simulink model "35-Bus_Network_Electricity_Transmission_Model"  (R2023b)
settings: Solver=VariableStepAuto  StartTime=0.0  StopTime=10  RelTol=1e-3
undefined symbols (not defined in the file): D1, D11, Delta
libraries: spsSeriesRLCBranchLib x47, spsLoadFlowBusLib x35, spsThreePhaseSeriesRLCLoadLib x27, spsDistributedParametersLineLib x22, spsGenericPowerSystemStabilizerLib x20, spsThreePhaseTransformerTwoWindingsLib x19, spsThreePhaseVIMeasurementLib x13, spsSynchronousMachinepuStandardLib x10, spsExcitationSystemLib x10, spsHydraulicTurbineandGovernorLib x10, spsThreePhaseParallelRLCLoadLib x4, spsGroundLib x3
(part 1 of 7)
settings Model: Creator=3.22  LastModifiedBy=3.22

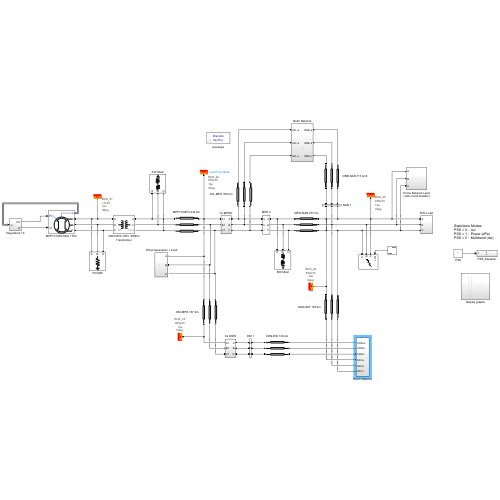
[thumbnail: Simulink's stored preview of the top-level diagram]
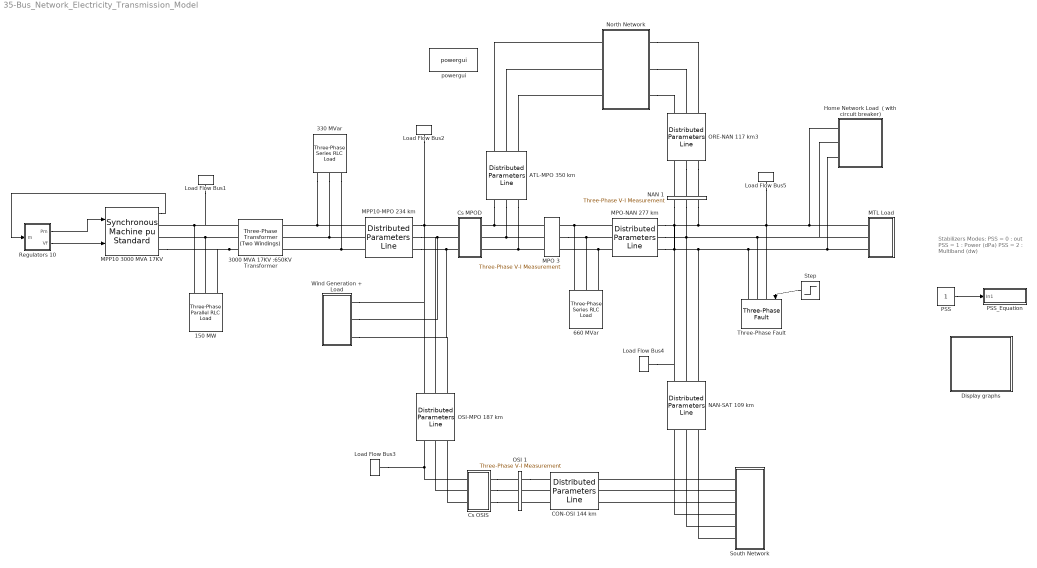
== system 35-Bus_Network_Electricity_Transmission_Model ==
  note: Stabilizers Modes:
      | PSS = 0 :  out
      | PSS = 1 :  Power (dPa)
      | PSS = 2 :  Multiband (dw)
  " Wind Generation + Load" : Subsystem
  150 MW : spsThreePhaseParallelRLCLoadLib/Three-Phase Parallel RLC Load  LConnTagsString=A|B|C  Configuration=Y (grounded)  NominalVoltage=1000  Vabc=[1e3 1e3 1e3]  Vabcp=[1e3 1e3 1e3]  NominalFrequency=60  UnbalancedPower=off  ActivePower=150e6  InductivePower=0  CapacitivePower=0  Pabc=[10e3 9e3 11e3]  QLabc=[100 90 110]  QCabc=[100 90 110]  Pabcp=[10e3 9e3 11e3]  QLabcp=[100 90 110]  QCabcp=[100 90 110]  Measurements=None  LoadType=constant Z
  "3000 MVA 17KV :650KV Transformer " : spsThreePhaseTransformerTwoWindingsLib/Three-Phase Transformer (Two Windings)  Winding1Connection=Delta (D1)  Winding2Connection=Yg  CoreType=Three single-phase transformers  SetSaturation=off  Hysteresis=off  DataFile='hysteresis'  SetInitialFlux=off  Measurements=None  UNITS=pu  NominalPower=[ 3000e6 , 60 ]  Winding1=[ 17e3 , 0.002 , 0.08 ]  Winding2=[ 650e3 , 0.002 , 0.08 ]  Rm=500  Lm=500  L0=0.5  Saturation=[ 0,0 ; 0.0024,1.2 ; 1.0,1.52 ]  InitialFluxes=[ 0.8 , -0.8 , 0.7 ]  BreakLoop=off  DiscreteSolver=Trapezoidal iterative  DataType=off  TransfoNumber=1
  330 MVar : spsThreePhaseSeriesRLCLoadLib/Three-Phase Series RLC Load  LConnTagsString=A|B|C  Configuration=Y (grounded)  NominalVoltage=1000  Vabc=[1e3 1e3 1e3]  Vabcp=[1e3 1e3 1e3]  NominalFrequency=60  UnbalancedPower=off  ActivePower=1100e3  InductivePower=330e6  CapacitivePower=0  Pabc=[10e3 9e3 11e3]  QLabc=[100 90 110]  QCabc=[100 90 110]  Pabcp=[10e3 9e3 11e3]  QLabcp=[100 90 110]  QCabcp=[100 90 110]  Measurements=None  LoadType=constant Z
  660 MVar : spsThreePhaseSeriesRLCLoadLib/Three-Phase Series RLC Load  LConnTagsString=A|B|C  Configuration=Y (grounded)  NominalVoltage=1000  Vabc=[1e3 1e3 1e3]  Vabcp=[1e3 1e3 1e3]  NominalFrequency=60  UnbalancedPower=off  ActivePower=2200e3  InductivePower=660e6  CapacitivePower=0  Pabc=[10e3 9e3 11e3]  QLabc=[100 90 110]  QCabc=[100 90 110]  Pabcp=[10e3 9e3 11e3]  QLabcp=[100 90 110]  QCabcp=[100 90 110]  Measurements=None  LoadType=constant Z
  ATL-MPO 350 km : spsDistributedParametersLineLib/Distributed Parameters Line  Phases=3  Length=350  Frequency=60  Resistance=[0.01273 0.3864]/6  Inductance="[0.9337e-3  4.1264e-3]/6"  Capacitance=[12.74e-9 7.751e-9]*6  x1=[-0.00198 6.98010668023183e-15 0.00211514985966667 -0.00384910891782008;-0.00192 6.88834857923299e-15 0.00223032100016454 -0.00383079412320694;-0.00186 6.79306627181897e-15 0.00234435106722713 -0.00381051942353543;-0.0018 6.69430850617886e-15 0.00245718172096511 -0.00378829519171654;-0.00174 6.59212580861038e-15 0.00256875523513113 -0.00376413279807792;-0.00168 6.48657045766974e-15 0.00267901452665373 -0.00373804460454662;-0.00162 6.37769645742491e-15 0.002787903184842 -0.00371004395832451;-0.00156 6.26555950982618e-15 0.00289536550024637 -0.0036801451850596;-0.0015 6.150216986208e-15 0.00300134649316061 -0.00364836358151674;-0.00144 6.03172789793673e-15 0.00310579194175044 -0.00361471540775158;-0.00138 5.91015286621936e-15 0.00320864840979444 -0.00357921787879154;-0.00132 5.78555409108856e-15 0.00330986327402298 -0.00354188915582838;-0.00126 5.65799531958002e-15 0.00340938475104129 -0.0035027483369265;-0.0012 5.52754181311824e-15 0.00350716192382279 -0.00346181544725211;-0.00114 5.39426031412764e-15 0.00360314476775915 -0.00341911142882791;-0.00108 5.25821901188587e-15 0.00369728417625386 -0.0033746581298188;-0.00102 5.1194875076369e-15 0.00378953198584605 -0.00332847829335396;-0.00096 4.97813677898177e-15 0.00387984100085178 -0.00328059554589104;-0.0009 4.83423914356512e-15 0.00396816501751025 -0.00323103438512841;-0.00084 4.68786822207615e-15 0.00405445884762251 -0.00317982016747169;-0.00078 4.53909890058292e-15 0.00413867834167054 -0.00312697909506097;-0.00072 4.38800729221925e-15 0.00422078041140498 -0.00307253820236529;-0.00066 4.23467069824383e-15 0.0043007230518899 -0.0030165253423513;-0.0006 4.07916756849147e-15 0.00437846536299324 -0.00295896917223319;-0.00054 3.92157746123672e-15 0.00445396757031214 -0.00289989913881109;-0.00048 3.76198100249039e-15 0.00452719104552221 -0.00283934546340561;-0.00042 3.60045984474976e-15 0.00459809832614052 -0.00277733912639597;-0.00036 3.43709662522371e-15 0.00466665313469209 -0.00271391185136995;-0.0003 3.27197492355395e-15 0.00473282039727011 -0.00264909608889343;-0.00024 3.10517921905415e-15 0.00479656626148042 -0.00258292499990818;-0.00018 2.93679484748877e-15 0.00485785811376101 -0.002515432438766;-0.00012 2.76690795741369e-15 0.0049166645960677 -0.0024466529359083;-6e-05 2.59560546610101e-15 0.00497295562191752 -0.00237662168019965]  x2=[-0.00198 9.14273446462953e-13 -0.141743524193211 -0.279232793755801;-0.00192 9.90097800622471e-13 -0.134363025534958 -0.282492907357275;-0.00186 1.06541560245229e-12 -0.126913784270099 -0.285608492367477;-0.0018 1.14018831797327e-12 -0.119399611568109 -0.288577954795545;-0.00174 1.21437769208252e-12 -0.11182435181859 -0.291399775409632;-0.00168 1.28794576812539e-12 -0.104191880664404 -0.294072510514171;-0.00162 1.36085490731478e-12 -0.0965061030188257 -0.296594792688496;-0.00156 1.43306780798787e-12 -0.0887709510677152 -0.29896533148644;-0.0015 1.50454752469036e-12 -0.0809903822577399 -0.301182914096551;-0.00144 1.57525748707837e-12 -0.0731683772716712 -0.30324640596259;-0.00138 1.64516151862858e-12 -0.0653089379917943 -0.305154751363989;-0.00132 1.71422385514677e-12 -0.0574160854524703 -0.306906973955978;-0.00126 1.78240916306545e-12 -0.0494938577829015 -0.308502177269103;-0.0012 1.84968255752117e-12 -0.0415463081411497 -0.309939545167873;-0.00114 1.91600962020226e-12 -0.0335775026404654 -0.31121834226831;-0.00108 1.98135641695787e-12 -0.0255915182689893 -0.312337914314189;-0.00102 2.0456895151593e-12 -0.0175924408038899 -0.313297688511763;-0.00096 2.10897600080479e-12 -0.00958436272100424 -0.31409717382282;-0.0009 2.17118349535886e-12 -0.0015713811010519 -0.3147359612159;-0.00084 2.23228017231786e-12 0.00644240446650752 -0.31521372387557;-0.00078 2.29223477349289e-12 0.0144528939809 -0.315530217369625;-0.00072 2.35101662500219e-12 0.0224559891276729 -0.315685279774147;-0.00066 2.40859565296433e-12 0.0304475953754693 -0.315678831756342;-0.0006 2.46494239888469e-12 0.0384236240708646 -0.315510876615137;-0.00054 2.52002803472689e-12 0.0463799945301984 -0.315181500279485;-0.00048 2.57382437766175e-12 0.0543126361273268 -0.314690871264405;-0.00042 2.62630390448619e-12 0.0622174903762302 -0.314039240584767;-0.00036 2.67743976570459e-12 0.0700905130074102 -0.313226941626869;-0.0003 2.72720579926545e-12 0.0779276760370118 -0.312254389977866;-0.00024 2.77557654394643e-12 0.085724969827615 -0.311122083213152;-0.00018 2.82252725238078e-12 0.093478405139639 -0.309830600641792;-0.00012 2.8680339037185e-12 0.101184015172311 -0.308380603010131;-6e-05 2.91207321591591e-12 0.108837857593156 -0.306772832163753]  x3=[-0.00198 -3.31408931648922e-14 -0.0161917965503002 0.00683182870242155;-0.00192 -3.27443580437374e-14 -0.0163349113753115 0.00651312629500997;-0.00186 -3.23310703039613e-14 -0.0164696689578288 0.00619109165183713;-0.0018 -3.19012413912081e-14 -0.0165960003533827 0.00586588953177699;-0.00174 -3.14550912138921e-14 -0.0167138409284971 0.00553768631424321;-0.00168 -3.09928480306878e-14 -0.0168231303937561 0.00520664991406639;-0.00162 -3.05147483337489e-14 -0.01692381283465 0.00487294969558571;-0.00156 -3.00210367277148e-14 -0.0170158367401816 0.004536756385999;-0.0015 -2.95119658045659e-14 -0.0170991550292203 0.0041982419880156;-0.00144 -2.89877960143928e-14 -0.0171737250745901 0.00385757969185654;-0.00138 -2.8448795532146e-14 -0.0172395087248778 0.00351494378664725;-0.00132 -2.78952401204316e-14 -0.0172964723239523 0.00317050957124801;-0.00126 -2.73274129884268e-14 -0.0173445867281838 0.00282445326456784;-0.0012 -2.67456046469846e-14 -0.0173838273213541 0.00247695191540763;-0.00114 -2.6150112760003e-14 -0.0174141740272506 0.00212818331187868;-0.00108 -2.55412419921349e-14 -0.0174356113199377 0.00177832589044307;-0.00102 -2.49193038529158e-14 -0.0174481282317006 0.00142755864462222;-0.00096 -2.42846165373897e-14 -0.0174517183586558 0.00107606103342054;-0.0009 -2.36375047633149e-14 -0.017446379864028 0.000724012889510833;-0.00084 -2.29782996050323e-14 -0.0174321154790897 0.000371594327228634;-0.00078 -2.23073383240817e-14 -0.0174089325017639 1.89856504223522e-05;-0.00072 -2.16249641966523e-14 -0.0173768427928901 -0.000333632739793501;-0.00066 -2.09315263379564e-14 -0.0173358627701563 -0.000686080437334852;-0.0006 -2.02273795236159e-14 -0.0172860133996994 -0.00103817712344715;-0.00054 -1.95128840081521e-14 -0.0172273201853784 -0.00138974265895979;-0.00048 -1.87884053406732e-14 -0.0171598131557262 -0.00174059717644861;-0.00042 -1.80543141778521e-14 -0.0170835268485868 -0.00209056117225943;-0.00036 -1.73109860942922e-14 -0.0169985002934443 -0.00243945559834538;-0.0003 -1.65588013903763e-14 -0.0169047769914555 -0.00278710195387127;-0.00024 -1.57981448976976e-14 -0.0168024048931935 -0.00313332237653783;-0.00018 -1.50294057821731e-14 -0.0166914363741154 -0.00347793973357942;-0.00012 -1.42529773449389e-14 -0.016571928207766 -0.00382077771238837;-6e-05 -1.34692568211303e-14 -0.0164439415367315 -0.0041616609107198]  x4=[-0.00198 2.98411089605461e-14 0.0114570231609346 -0.0122817125842966;-0.00192 3.00466879551929e-14 0.0117485485103798 -0.0120667412107585;-0.00186 3.02368945090828e-14 0.0120340630853189 -0.0118455962694493;-0.0018 3.04116313090283e-14 0.0123134208112197 -0.0116183909022071;-0.00174 3.05708089564538e-14 0.0125864787635076 -0.0113852413514962;-0.00168 3.07143460131335e-14 0.0128530972406887 -0.0111462669009348;-0.00162 3.08421690428571e-14 0.0131131398358235 -0.0109015898142675;-0.00156 3.09542126490005e-14 0.0133664735063153 -0.010651335272813;-0.0015 3.10504195079847e-14 0.0136129686419773 -0.010395631311419;-0.00144 3.11307403986028e-14 0.0138524991313433 -0.0101346087529568;-0.00138 3.1195134227203e-14 0.014084942426189 -0.00986840114139055;-0.00132 3.12435680487128e-14 0.0143101796042296 -0.00959714467345329;-0.00126 3.12760170834941e-14 0.014528095429963 -0.00932097812896625;-0.0012 3.12924647300211e-14 0.014738578413626 -0.00904004279983656;-0.00114 3.1292902573374e-14 0.0149415208682351 -0.00875448241776969;-0.00108 3.1277330389544e-14 0.0151368189646803 -0.00846444308073365;-0.00102 3.12457561455481e-14 0.015324372784847 -0.00817007317821258;-0.00096 3.11981959953529e-14 0.0155040863727352 -0.00787152331528794;-0.0009 3.11346742716102e-14 0.0156758677835524 -0.00756894623558618;-0.00084 3.10552234732074e-14 0.0158396291307549 -0.00726249674313224;-0.00078 3.09598842486412e-14 0.0159952866310113 -0.00695233162314901;-0.00072 3.08487053752205e-14 0.0161427606470684 -0.00663860956184305;-0.00066 3.07217437341113e-14 0.0162819757284946 -0.00632149106521786;-0.0006 3.05790642812352e-14 0.0164128606502817 -0.00600113837695597;-0.00054 3.04207400140367e-14 0.0165353484492854 -0.00567771539541215;-0.00048 3.02468519341363e-14 0.0166493764584843 -0.00535138758975991;-0.00042 3.00574890058889e-14 0.0167548863390419 -0.00502232191533449;-0.00036 2.98527481108675e-14 0.0168518241101538 -0.00469068672821533;-0.0003 2.96327339982972e-14 0.016940140176665 -0.0043566516990921;-0.00024 2.93975592314635e-14 0.0170197893544441 -0.00402038772645795;-0.00018 2.91473441301224e-14 0.0170907308934998 -0.00368206684917471;-0.00012 2.88822167089435e-14 0.0171529284988301 -0.00334186215845466;-6e-05 2.86023126120142e-14 0.0172063503489906 -0.00299994770930384]  x5=0.0019793954844851  V1=[4.219e-16 0.0001256 0.0001256;377 377 377;2.896 1.02 -0.5506]  V2=[3.447e-16 8.016e-05 8.016e-05;377 377 377;2.788 1.015 -0.5555]  I1=[4.128e-19 5.188e-07 5.188e-07;377 377 377;2.697 1.572 0.0007381]  I2=[5.884e-19 5.436e-07 5.436e-07;377 377 377;2.289 0.05248 -1.518]  nHarmo=1  Measurements=None  Decoupling=off  VsMag0=0  VrMag0=0  VsAngle0=0  VrAngle0=0  IsMag0=0  IrMag0=0  IsAngle0=0  IrAngle0=0
      settings: LibrarySourceBlock=sps_lib/Power Grid Elements/Distributed Parameters Line
  CON-OSI 144 km : spsDistributedParametersLineLib/Distributed Parameters Line  Phases=3  Length=144  Frequency=60  Resistance=[0.01273 0.3864]/6  Inductance="[0.9337e-3  4.1264e-3]/6"  Capacitance=[12.74e-9 7.751e-9]*6  x1=[-0.00084 -6.12106331906545e-12 0 0;-0.00078 -5.96931950471425e-12 0 0;-0.00072 -5.8145216762041e-12 0 0;-0.00066 -5.65674903096439e-12 0 0;-0.0006 -5.49608228839574e-12 0 0;-0.00054 -5.33260364857242e-12 -13.3263292704613 8.49263982125866;-0.00048 -5.1663967501873e-12 -13.5399966121397 8.3110034847415;-0.00042 -4.99754662776075e-12 -13.7467366413609 8.12511508527185;-0.00036 -4.8261396681354e-12 -13.9464435861059 7.93506972678971;-0.0003 -4.65226356627902e-12 -14.1390152726117 7.74096464001211;-0.00024 -4.47600728041818e-12 -14.324353177645 7.54289913268811;-0.00018 -4.29746098652558e-12 -14.5023624789089 7.34097453879107;-0.00012 -4.11671603218432e-12 -14.6729521035559 7.13529416667437;-6e-05 -3.93386488985283e-12 -14.8360347747817 6.92596324621692]  x2=[-0.00084 -4.40472411926851e-12 0 0;-0.00078 -4.29950048512916e-12 0 0;-0.00072 -4.19207714709598e-12 0 0;-0.00066 -4.08250906493367e-12 0 0;-0.0006 -3.97085229569764e-12 0 0;-0.00054 -3.85716396505422e-12 -8.94549366124329 5.71026905715697;-0.00048 -3.74150223805408e-12 -9.08922753957406 5.58838070697636;-0.00042 -3.62392628937395e-12 -9.22831120114597 5.46363323796466;-0.00036 -3.50449627304171e-12 -9.36267348818779 5.33609047323209;-0.0003 -3.38327329166053e-12 -9.49224565847074 5.20581766601379;-0.00024 -3.26031936514764e-12 -9.61696142047828 5.07288146628511;-0.00018 -3.13569739900377e-12 -9.73675696732208 4.93734988666221;-0.00012 -3.00947115212954e-12 -9.85157100938683 4.79929226760556;-6e-05 -2.88170520420524e-12 -9.96134480568707 4.65877924194407]  x3=[-0.00084 5.02734058306821e-15 0 0;-0.00078 6.70201184862852e-15 0 0;-0.00072 8.37325424108812e-15 0 0;-0.00066 1.0040212721958e-14 0 0;-0.0006 1.17020344444776e-14 0 0;-0.00054 1.33578691899466e-14 -0.627617797454106 -0.11745005126189;-0.00048 1.50068698027131e-14 -0.620824228506745 -0.128185682906486;-0.00042 1.66481926235933e-14 -0.613713034412567 -0.138855732387108;-0.00036 1.82809979215042e-14 -0.60628785338987 -0.149454740709282;-0.0003 1.99044503230843e-14 -0.598552484298468 -0.159977285224503;-0.00024 2.15177192400873e-14 -0.59051088469612 -0.170417982404563;-0.00018 2.31199792943252e-14 -0.582167168813775 -0.180771490595862;-0.00012 2.47104107399481e-14 -0.573525605450653 -0.191032512752299;-6e-05 2.62881998828405e-14 -0.564590615790247 -0.201195799145338]  x4=[-0.00084 -1.00461865876865e-13 0 0;-0.00078 -1.00433753021638e-13 0 0;-0.00072 -1.00354256402562e-13 0 0;-0.00066 -1.00223416691577e-13 0 0;-0.0006 -1.00041300828697e-13 0 0;-0.00054 -9.98080019877624e-14 0.169804112382748 0.458131219894259;-0.00048 -9.95236395287709e-14 0.15407641971246 0.462833113851965;-0.00042 -9.91883589368111e-14 0.138269898698842 0.467298213836452;-0.00036 -9.8802331747629e-14 0.122392636250115 0.471524235420061;-0.0003 -9.83657554598677e-14 0.106452755467127 0.475509016492064;-0.00024 -9.78788534340229e-14 0.0904584114874216 0.479250518364833;-0.00018 -9.73418747781681e-14 0.0744177873129197 0.482746826816875;-0.00012 -9.67550942205056e-14 0.0583390896233459 0.485996153072182;-6e-05 -9.61188119688114e-14 0.0422305445775383 0.488996834715401]  x5=0.000814379856473869  V1=[3.066e-13 0.3294 0.3294;377 377 377;-0.5534 -1.851 2.861]  V2=[2.167e-13 0.2213 0.2213;377 377 377;-0.5727 -1.852 2.86]  I1=[4.19e-16 0.002316 0.002316;377 377 377;0.2564 -0.79 -2.361]  I2=[5.677e-16 0.002387 0.002387;377 377 377;-1.374 -3.038 1.674]  nHarmo=1  Measurements=None  Decoupling=off  VsMag0=0  VrMag0=0  VsAngle0=0  VrAngle0=0  IsMag0=0  IrMag0=0  IsAngle0=0  IrAngle0=0
      settings: LibrarySourceBlock=sps_lib/Power Grid Elements/Distributed Parameters Line
  Cs MPOD : Subsystem
  Cs OSIS : Subsystem
  Display graphs : Subsystem
  Home Network Load （with circuit breaker) : Subsystem
  Load Flow Bus1 : spsLoadFlowBusLib/Load Flow Bus  LConnTagsString=a  Phases=single  Connectors=on one side  ID=BUS_21  Vbase=17e3  Vref=1  Vangle=0  VLF=1  VLFb=1  VLFc=1  angleLF=0  angleLFb=0  angleLFc=0
  Load Flow Bus2 : spsLoadFlowBusLib/Load Flow Bus  LConnTagsString=a  Phases=single  Connectors=on one side  ID=BUS_22  Vbase=650e3  Vref=1  Vangle=0  VLF=1  VLFb=1  VLFc=1  angleLF=0  angleLFb=0  angleLFc=0
  Load Flow Bus3 : spsLoadFlowBusLib/Load Flow Bus  LConnTagsString=a  Phases=single  Connectors=on one side  ID=BUS_23  Vbase=650e3  Vref=1  Vangle=0  VLF=1  VLFb=1  VLFc=1  angleLF=0  angleLFb=0  angleLFc=0
  Load Flow Bus4 : spsLoadFlowBusLib/Load Flow Bus  LConnTagsString=a  Phases=single  Connectors=on one side  ID=BUS_24  Vbase=650e3  Vref=1  Vangle=0  VLF=1  VLFb=1  VLFc=1  angleLF=0  angleLFb=0  angleLFc=0
  Load Flow Bus5 : spsLoadFlowBusLib/Load Flow Bus  LConnTagsString=a  Phases=single  Connectors=on one side  ID=BUS_25  Vbase=650e3  Vref=1  Vangle=0  VLF=1  VLFb=1  VLFc=1  angleLF=0  angleLFb=0  angleLFc=0
  MPO 3 : spsThreePhaseVIMeasurementLib/Three-Phase V-I Measurement  VoltageMeasurement=no  SetLabelV=off  LabelV=Vabc_MPO3  Vpu=off  VpuLL=off  CurrentMeasurement=no  SetLabelI=off  LabelI=Iabc  Ipu=off  Pbase=100e6  Vbase=500e3  OutputType=Complex  PhasorSimulation=off  PSBequivalent=0
  MPO-NAN 277 km : spsDistributedParametersLineLib/Distributed Parameters Line  Phases=3  Length=277  Frequency=60  Resistance=[0.01273 0.3864]/6  Inductance="[0.9337e-3  4.1264e-3]/6"  Capacitance=[12.74e-9 7.751e-9]*6  x1=[-0.00162 6.37769645742491e-15 0.002787903184842 -0.00371004395832451;-0.00156 6.26555950982618e-15 0.00289536550024637 -0.0036801451850596;-0.0015 6.150216986208e-15 0.00300134649316061 -0.00364836358151674;-0.00144 6.03172789793673e-15 0.00310579194175044 -0.00361471540775158;-0.00138 5.91015286621936e-15 0.00320864840979444 -0.00357921787879154;-0.00132 5.78555409108856e-15 0.00330986327402298 -0.00354188915582838;-0.00126 5.65799531958002e-15 0.00340938475104129 -0.0035027483369265;-0.0012 5.52754181311824e-15 0.00350716192382279 -0.00346181544725211;-0.00114 5.39426031412764e-15 0.00360314476775915 -0.00341911142882791;-0.00108 5.25821901188587e-15 0.00369728417625386 -0.0033746581298188;-0.00102 5.1194875076369e-15 0.00378953198584605 -0.00332847829335396;-0.00096 4.97813677898177e-15 0.00387984100085178 -0.00328059554589104;-0.0009 4.83423914356512e-15 0.00396816501751025 -0.00323103438512841;-0.00084 4.68786822207615e-15 0.00405445884762251 -0.00317982016747169;-0.00078 4.53909890058292e-15 0.00413867834167054 -0.00312697909506097;-0.00072 4.38800729221925e-15 0.00422078041140498 -0.00307253820236529;-0.00066 4.23467069824383e-15 0.0043007230518899 -0.0030165253423513;-0.0006 4.07916756849147e-15 0.00437846536299324 -0.00295896917223319;-0.00054 3.92157746123672e-15 0.00445396757031214 -0.00289989913881109;-0.00048 3.76198100249039e-15 0.00452719104552221 -0.00283934546340561;-0.00042 3.60045984474976e-15 0.00459809832614052 -0.00277733912639597;-0.00036 3.43709662522371e-15 0.00466665313469209 -0.00271391185136995;-0.0003 3.27197492355395e-15 0.00473282039727011 -0.00264909608889343;-0.00024 3.10517921905415e-15 0.00479656626148042 -0.00258292499990818;-0.00018 2.93679484748877e-15 0.00485785811376101 -0.002515432438766;-0.00012 2.76690795741369e-15 0.0049166645960677 -0.0024466529359083;-6e-05 2.59560546610101e-15 0.00497295562191752 -0.00237662168019965]  x2=[-0.00162 3.45357352044025e-13 -0.0116853448372484 -0.0542657161926271;-0.00156 2.87134243606378e-13 -0.0102864722355918 -0.0545635202751054;-0.0015 2.28764231984071e-13 -0.00888233688466737 -0.054833408652393;-0.00144 1.70277180353604e-13 -0.00747365716606598 -0.0550752432446092;-0.00138 1.11703011771307e-13 -0.00606115378636113 -0.0552889003247079;-0.00132 5.30716938641543e-14 -0.00464554940838193 -0.0554742705817792;-0.00126 -5.58677650223161e-15 -0.00322756828148552 -0.055631259176974;-0.0012 -6.42423885705273e-14 -0.0018079358710177 -0.0557597857920265;-0.00114 -1.22865133045767e-13 -0.000387378487151455 -0.0558597846703454;-0.00108 -1.81425017448655e-13 0.00103337708670675 -0.0559312046506569;-0.00102 -2.39892081460267e-13 0.00245360396575279 -0.0559740091931792;-0.00096 -2.98236412250307e-13 0.00387257553567255 -0.0559881763983175;-0.0009 -3.56428159781065e-13 0.00528956582439131 -0.0559736990178678;-0.00084 -4.14437552079244e-13 0.00670384987349436 -0.0559305844587256;-0.00078 -4.72234910467854e-13 0.00811470410912923 -0.055858854779096;-0.00072 -5.2979066475037e-13 0.00952140671219937 -0.0557585466772083;-0.00066 -5.87075368339395e-13 0.0109232379876602 -0.0556297114725412;-0.0006 -6.44059713322071e-13 0.0123194807327283 -0.0554724150795658;-0.00054 -7.00714545454557e-13 0.0137094206038157 -0.0552867379740233;-0.00048 -7.57010879077872e-13 0.0150923464820012 -0.0550727751517519;-0.00042 -8.12919911947498e-13 0.0164675508368521 -0.0548306360800849;-0.00036 -8.68413039969138e-13 0.0178343300884094 -0.0545604446418457;-0.0003 -9.23461871833103e-13 0.019191984967153 -0.0542623390719667;-0.00024 -9.78038243539824e-13 0.0205398208717603 -0.0539364718867656;-0.00018 -1.03211423280908e-12 0.0218771482244773 -0.0535830098059159;-0.00012 -1.08566217336556e-12 0.0232032828239195 -0.0532021336671493;-6e-05 -1.13865466909341e-12 0.0245175461951216 -0.0527940383337362]  x3=[-0.00162 3.43834216329146e-14 -0.0035424404892329 0.000742255688742989;-0.00156 3.43011259819442e-14 -0.00355650736100562 0.000670266158361229;-0.0015 3.42012812411094e-14 -0.00356875465789576 0.000597933707427756;-0.00144 3.40839384928247e-14 -0.00357917611395991 0.000525295342561018;-0.00138 3.39491577718082e-14 -0.00358776639738859 0.000452388226890684;-0.00132 3.37970080343674e-14 -0.00359452111323406 0.0003792496610443;-0.00126 3.36275671231193e-14 -0.0035994368056589 0.000305917064063598;-0.0012 3.34409217271651e-14 -0.00360251095970401 0.000232427954260223;-0.00114 3.3237167337738e-14 -0.00360374200257538 0.000158819930020674;-0.00108 3.30164081993487e-14 -0.00360312930444875 8.51306505702711e-05;-0.00102 3.27787572564515e-14 -0.00360067317879178 1.13978167060029e-05;-0.00096 3.25243360956602e-14 -0.00359637488220375 -6.23408484918991e-05;-0.0009 3.22532748835416e-14 -0.00359023661377262 -0.000136047618959787;-0.00084 3.19657123000207e-14 -0.00358226151394994 -0.000209684784951943;-0.00078 3.16617954674286e-14 -0.00357245366294414 -0.000283214672333589;-0.00072 3.13416798752327e-14 -0.00356081807863303 -0.000356599661855663;-0.00066 3.10055293004849e-14 -0.00354736071399653 -0.000429802208401528;-0.0006 3.06535157240307e-14 -0.00353208845407106 -0.000502784860195743;-0.00054 3.02858192425202e-14 -0.003515009112427 -0.000575510277965086;-0.00048 2.99026279762677e-14 -0.00349613142717112 -0.000647941254042015;-0.00042 2.95041379730054e-14 -0.00347546505647602 -0.000720040731400798;-0.00036 2.90905531075824e-14 -0.00345302057363882 -0.000791771822616573;-0.0003 2.8662084977658e-14 -0.00342880946167165 -0.000863097828737637;-0.00024 2.82189527954445e-14 -0.00340284410742679 -0.000933982258061304;-0.00018 2.77613832755546e-14 -0.00337513779525923 -0.00100438884480374;-0.00012 2.72896105190095e-14 -0.00334570470023024 -0.0010742815676542;-6e-05 2.68038758934689e-14 -0.0033145598808551 -0.00114362466820421]  x4=[-0.00162 -2.58146661290416e-14 0.00308060475276878 -0.00196444936876967;-0.00156 -2.61439083122915e-14 0.00312699034413802 -0.00190360844875017;-0.0015 -2.6459774788965e-14 0.00317177610946707 -0.00184179360747365;-0.00144 -2.67621039559361e-14 0.00321493913553082 -0.00177903647055511;-0.00138 -2.70507411360165e-14 0.0032564573393276 -0.00171536914570542;-0.00132 -2.73255386570914e-14 0.00329630947937716 -0.00165082420630441;-0.00126 -2.75863559276715e-14 0.00333447516658827 -0.00158543467473573;-0.0012 -2.78330595088218e-14 0.00337093487469015 -0.001519234005492;-0.00114 -2.80655231824315e-14 0.00340566995022241 -0.00145225606805883;-0.00108 -2.82836280157899e-14 0.0034386626220786 -0.00138453512958664;-0.00102 -2.8487262422434e-14 0.00346989601059815 -0.00131610583735889;-0.00096 -2.86763222192387e-14 0.00349935413620237 -0.0012470032010659;-0.0009 -2.88507106797186e-14 0.00352702192756989 -0.00117726257489328;-0.00084 -2.90103385835148e-14 0.00355288522934738 -0.00110691963943403;-0.00078 -2.91551242620423e-14 0.00357693080939177 -0.00103601038343372;-0.00072 -2.92849936402726e-14 0.00359914636554 -0.000964571085377981;-0.00066 -2.93998802746321e-14 0.00361952053190303 -0.000892638294931735;-0.0006 -2.94997253869958e-14 0.0036380428846809 -0.000820248814239743;-0.00054 -2.95844778947591e-14 0.00365470394749565 -0.00074743967909793;-0.00048 -2.96540944369733e-14 0.00366949519623971 -0.000674248140005193;-0.00042 -2.97085393965288e-14 0.00368240906343689 -0.000600711643105357;-0.00036 -2.97477849183784e-14 0.00369343894211412 -0.000526867811029033;-0.0003 -2.97718109237878e-14 0.00370257918918167 -0.000452754423645189;-0.00024 -2.97806051206089e-14 0.00370982512832023 -0.000378409398732268;-0.00018 -2.97741630095679e-14 0.00371517305237345 -0.000303870772578754;-0.00012 -2.9752487886568e-14 0.00371862022524458 -0.000229176680523103;-6e-05 -2.97155908410025e-14 0.00372016488329627 -0.000154365337442997]  x5=0.00156655014057821  V1=[4.219e-16 0.0001256 0.0001256;377 377 377;3.052 1.115 -0.4557]  V2=[4.095e-15 0.006804 0.006804;377 377 377;-1.109 1.061 -0.5096]  I1=[9.849e-18 6.958e-05 6.958e-05;377 377 377;-2.423 -0.4689 -2.04]  I2=[7.867e-18 6.871e-05 6.871e-05;377 377 377;0.191 2.298 0.7273]  nHarmo=1  Measurements=None  Decoupling=off  VsMag0=0  VrMag0=0  VsAngle0=0  VrAngle0=0  IsMag0=0  IrMag0=0  IsAngle0=0  IrAngle0=0
      settings: LibrarySourceBlock=sps_lib/Power Grid Elements/Distributed Parameters Line
  MPP10 3000 MVA 17KV : spsSynchronousMachinepuStandardLib/Synchronous Machine pu Standard  PresetModel=No  MechanicalLoad=Mechanical power Pm  ShowDetailedParameters=on  RotorType=Salient-pole  Units=per unit standard parameters  MeasurementBus=off  NominalParameters="[3000e6  17000   60]"  Reactances1=[ 1.81, 0.3, 0.23, 1.76, 0.65, 0.25, 0.15 ]  Reactances2=[2.24 0.17 0.12 1.02 0.13 0.08]  dAxisTimeConstants=Short-circuit  qAxisTimeConstants=Open-circuit  TimeConstants1="[ 4.4849  0.0681  0.1  ]"  TimeConstants2=[ 8.0, 0.03, 1.0, 0.07 ]  TimeConstants3="[  4.49  0.0681  0.0513  ]"  TimeConstants4=[ 8.0, 0.03, 0.3371, 0.0295 ]  TimeConstants5=[ 1.01, 0.053, 0.1 ]  TimeConstants6=[ 1.3201, 0.023, 1.0, 0.07 ]  TimeConstants7=[0.012 0.003 0.003]  TimeConstants8=[ 1.3201, 0.0231, 0.3371, 0.0295 ]  StatorResistance=0.037875  Mechanical=[3.8 0 28]  PolePairs=20  InitialConditions=[ 0 -107.876 0.604539 0.604539 0.604539 -42.1129 -162.113 77.8871 1.28555 ]  SetSaturation=off  Saturation=[0.6404,0.7127,0.8441,0.9214,0.9956,1.082,1.19,1.316,1.457;0.7,0.7698,0.8872,0.9466,0.9969,1.046,1.1,1.151,1.201]  LoadFlowParameters=[1,0,0,0,0]  TsPowergui=0  TsBlock=-1  IterativeModel=Trapezoidal non iterative  IterativeDiscreteModel=Trapezoidal non iterative  BusType=PV  Pref=2300e6  Qref=0  Qmin=-inf  Qmax=inf  PLF=0  QLF=0
  MPP10-MPO 234 km : spsDistributedParametersLineLib/Distributed Parameters Line  Phases=3  Length=234  Frequency=60  Resistance=[0.01273 0.3864]/6  Inductance="[0.9337e-3  4.1264e-3]/6"  Capacitance=[12.74e-9 7.751e-9]*6  x1=[-0.00138 2.70565629857601e-11 1.07097252173756 -3.44845409203551;-0.00132 2.64632447283607e-11 1.18045735649416 -3.4524056782375;-0.00126 2.58563873859737e-11 1.28933824745482 -3.45459094990138;-0.0012 2.52363014380289e-11 1.39755948914386 -3.45500878900179;-0.00114 2.46033041319553e-11 1.50506571357432 -3.45365898176453;-0.00108 2.39577193208709e-11 1.6118019185753 -3.45054221877591;-0.00102 2.32998772978942e-11 1.71771349593207 -3.44566009462948;-0.00096 2.26301146271597e-11 1.82274625932461 -3.43901510711016;-0.0009 2.19487739716255e-11 1.92684647205041 -3.43061065591635;-0.00084 2.12562039177606e-11 2.02996087451708 -3.42045104092057;-0.00078 2.0552758797202e-11 2.13203671149098 -3.40854145996959;-0.00072 1.98387985054714e-11 2.23302175908777 -3.39488800622509;-0.00066 1.91146883178466e-11 2.33286435149112 -3.37949766504629;-0.0006 1.83807987024795e-11 2.43151340738587 -3.3623783104161;-0.00054 1.76375051308581e-11 2.52891845609219 -3.34353870091271;-0.00048 1.68851878857082e-11 2.62502966338734 -3.32298847522843;-0.00042 1.61242318664335e-11 2.71979785700173 -3.30073814723846;-0.00036 1.53550263921944e-11 2.81317455177639 -3.27679910062174;-0.0003 1.45779650027248e-11 2.90511197446887 -3.25118358303685;-0.00024 1.379344525699e-11 2.99556308819492 -3.22390469985591;-0.00018 1.30018685297881e-11 3.0844816164934 -3.19497640745962;-0.00012 1.22036398063995e-11 3.17182206700222 -3.16441350609689;-6e-05 1.13991674753886e-11 3.25753975473303 -3.13223163231281]  x2=[-0.00138 -8.65543103929743e-12 -11.3616240421163 12.4769698760863;-0.00132 -8.50200366804866e-12 -11.7143796266815 12.3441892266905;-0.00126 -8.34422651462434e-12 -12.061141918173 12.2050930619919;-0.0012 -8.18218030073156e-12 -12.4017335065948 12.0597525461585;-0.00114 -8.01594793220763e-12 -12.7359801389969 11.908242038084;-0.00108 -7.84561445660388e-12 -13.0637108086261 11.7506390533438;-0.00102 -7.67126701967385e-12 -13.384757842416 11.587024224537;-0.00096 -7.49299482078784e-12 -13.6989569867718 11.4174812600333;-0.0009 -7.31088906729689e-12 -14.0061474916055 11.2420969011463;-0.00084 -7.12504292786941e-12 -14.3061721925787 11.0609608777545;-0.00078 -6.93555148482438e-12 -14.5988775915105 10.8741658623946;-0.00072 -6.74251168548546e-12 -14.8841139349102 10.6818074228481;-0.00066 -6.54602229258095e-12 -15.1617352905941 10.4839839732469;-0.0006 -6.34618383371497e-12 -15.4315996223466 10.2807967237232;-0.00054 -6.14309854993566e-12 -15.6935688625891 10.0723496286284;-0.00048 -5.9368703434268e-12 -15.9475089830177 9.85874933334797;-0.00042 -5.7276047243495e-12 -16.1932900631746 9.64010511973986;-0.00036 -5.51540875686124e-12 -16.4307863569175 9.41652885022383;-0.0003 -5.30039100433995e-12 -16.6598763567542 9.18813491055058;-0.00024 -5.08266147384086e-12 -16.8804428560076 8.95504015127987;-0.00018 -4.86233155981498e-12 -17.0923730087812 8.71736382799765;-0.00012 -4.63951398711753e-12 -17.2955583876928 8.47522754030267;-6e-05 -4.41432275333592e-12 -17.4898950393481 8.22875516959387]  x3=[-0.00138 -3.72430274266343e-13 1.48681909924038 0.371734732614772;-0.00132 -3.85202426918902e-13 1.46705787960671 0.397412025036263;-0.00126 -3.97777502892126e-13 1.44654608605372 0.422885994122415;-0.0012 -4.10149068544788e-13 1.425294212794 0.448143606919939;-0.00114 -4.22310794355298e-13 1.40331313267862 0.473171941167422;-0.00108 -4.34256458160011e-13 1.3806140916343 0.497958191906591;-0.00102 -4.45979948336592e-13 1.3572087029099 0.522489678033571;-0.00096 -4.57475266930842e-13 1.33310894113475 0.54675384878677;-0.0009 -4.68736532725359e-13 1.30832713619229 0.570738290168081;-0.00084 -4.79757984248478e-13 1.28287596691186 0.59443073129411;-0.00078 -4.90533982721948e-13 1.25676845458192 0.617819050674192;-0.00072 -5.01059014945832e-13 1.23001795628822 0.640891282411966;-0.00066 -5.11327696119163e-13 1.20263815807995 0.663635622327348;-0.0006 -5.2133477259491e-13 1.17464306796782 0.686040433995771;-0.00054 -5.31075124567838e-13 1.14604700875721 0.708094254701593;-0.00048 -5.40543768693897e-13 1.1168646107204 0.729785801302631;-0.00042 -5.49735860639793e-13 1.08711080411146 0.751103976002832;-0.00036 -5.58646697561434e-13 1.05680081152764 0.772037872030105;-0.0003 -5.67271720509998e-13 1.02595014012121 0.792576779216427;-0.00024 -5.75606516764374e-13 0.994574573665711 0.812710189477367;-0.00018 -5.83646822088787e-13 0.962690164480702 0.832427802188212;-0.00012 -5.91388522914467e-13 0.930313225219076 0.851719529453961;-6e-05 -5.98827658444219e-13 0.897460320521216 0.870575501270474]  x4=[-0.00138 5.47927057792979e-13 -1.67626482985383 -0.1532069712362;-0.00132 5.58217241869159e-13 -1.66264653750453 -0.181204688115209;-0.00126 5.68221831689729e-13 -1.64817760446446 -0.2091096973275;-0.0012 5.77935708721675e-13 -1.63286543330713 -0.236907722154735;-0.00114 5.87353903166015e-13 -1.61671785802224 -0.264584540613765;-0.00108 5.96471596500443e-13 -1.59974314000767 -0.292125992732857;-0.00102 6.05284123944573e-13 -1.58194996384282 -0.319517987796198;-0.00096 6.13786976846528e-13 -1.56334743284539 -0.34674651155297;-0.0009 6.2197580498965e-13 -1.54394506441398 -0.373797633387292;-0.00084 6.29846418818147e-13 -1.52375278515879 -0.400657513445387;-0.00078 6.37394791580554e-13 -1.502780925823 -0.427312409716304;-0.00072 6.44617061389886e-13 -1.48104021599735 -0.453748685062584;-0.00066 6.51509533199457e-13 -1.45854177863073 -0.479952814197275;-0.0006 6.58068680693332e-13 -1.43529712433941 -0.505911390603714;-0.00054 6.64291148090452e-13 -1.41131814551803 -0.531611133394552;-0.00048 6.7017375186152e-13 -1.38661711025525 -0.557038894106502;-0.00042 6.75713482357749e-13 -1.36120665605712 -0.582181663427331;-0.00036 6.80907505350655e-13 -1.33509978338154 -0.607026577851671;-0.0003 6.85753163482098e-13 -1.30830984898698 -0.63156092626222;-0.00024 6.90247977623843e-13 -1.28085055909889 -0.65577215643299;-0.00018 6.94389648145919e-13 -1.25273596239737 -0.679647881451252;-0.00012 6.98176056093158e-13 -1.22398044282959 -0.703175886054914;-6e-05 7.0160526426929e-13 -1.19459871225069 -0.726344132882075]  x5=0.00132336726677004  V1=[5.094e-16 1.649e-05 1.649e-05;377 377 377;1.389 -1.935 2.777]  V2=[3.793e-13 0.4417 0.4417;377 377 377;-0.7025 -1.967 2.745]  I1=[9.917e-16 0.005412 0.005412;377 377 377;-2.043 2.781 1.21]  I2=[8.773e-16 0.005353 0.005353;377 377 377;0.5828 -0.6661 -2.237]  nHarmo=1  Measurements=None  Decoupling=off  VsMag0=0  VrMag0=0  VsAngle0=0  VrAngle0=0  IsMag0=0  IrMag0=0  IsAngle0=0  IrAngle0=0
      settings: LibrarySourceBlock=sps_lib/Power Grid Elements/Distributed Parameters Line
  MTL Load : Subsystem
  NAN 1 : spsThreePhaseVIMeasurementLib/Three-Phase V-I Measurement  VoltageMeasurement=no  SetLabelV=off  LabelV=Vabc  Vpu=off  VpuLL=off  CurrentMeasurement=no  SetLabelI=off  LabelI=Iabc  Ipu=off  Pbase=100e6  Vbase=500e3  OutputType=Complex  PhasorSimulation=off  PSBequivalent=0
  NAN-SAT 109 km : spsDistributedParametersLineLib/Distributed Parameters Line  Phases=3  Length=109  Frequency=60  Resistance=[0.01273 0.3864]/6  Inductance="[0.9337e-3  4.1264e-3]/6"  Capacitance=[12.74e-9 7.751e-9]*6  x1=[-0.00066 8.33557454077081e-16 0 0;-0.0006 8.41338452335436e-16 0 0;-0.00054 8.48689006295428e-16 0 0;-0.00048 8.5560535527783e-16 0 0;-0.00042 8.62083960750703e-16 -0.000241694105416429 0.000278970692701831;-0.00036 8.68121508139775e-16 -0.000250270156684541 0.000277799813445786;-0.0003 8.73714908524242e-16 -0.000258718165116033 0.000276486806672031;-0.00024 8.78861300217113e-16 -0.00026703380855369 0.000275032344139095;-0.00018 8.83558050229303e-16 -0.000275212832560673 0.000273437169976883;-0.00012 8.8780275561672e-16 -0.000283251052597169 0.000271702100305974;-6e-05 8.91593244709655e-16 -0.000291144356161279 0.00026982802282007]  x2=[-0.00066 -5.87075368339395e-13 0 0;-0.0006 -6.44059713322071e-13 0 0;-0.00054 -7.00714545454557e-13 0 0;-0.00048 -7.57010879077872e-13 0 0;-0.00042 -8.12919911947498e-13 0.0164675508368521 -0.0548306360800849;-0.00036 -8.68413039969138e-13 0.0178343300884094 -0.0545604446418457;-0.0003 -9.23461871833103e-13 0.019191984967153 -0.0542623390719667;-0.00024 -9.78038243539824e-13 0.0205398208717603 -0.0539364718867656;-0.00018 -1.03211423280908e-12 0.0218771482244773 -0.0535830098059159;-0.00012 -1.08566217336556e-12 0.0232032828239195 -0.0532021336671493;-6e-05 -1.13865466909341e-12 0.0245175461951216 -0.0527940383337362]  x3=[-0.00066 7.78993735177572e-14 0 0;-0.0006 7.69861287196129e-14 0 0;-0.00054 7.60334963954755e-14 0 0;-0.00048 7.50419639296447e-14 0 0;-0.00042 7.40120386084514e-14 -0.00944479406674045 -0.00208183610746204;-0.00036 7.29442473607209e-14 -0.00937574164931692 -0.00227469078344568;-0.0003 7.18391364881858e-14 -0.00930189242922181 -0.00246638168559305;-0.00024 7.06972713859888e-14 -0.0092232841890807 -0.00265681074129658;-0.00018 6.95192362534154e-14 -0.00913995714632175 -0.00284588052353264;-0.00012 6.83056337950069e-14 -0.00905195393259976 -0.00303349430070704;-6e-05 6.70570849122059e-14 -0.00895931957198498 -0.00321955608614467]  x4=[-0.00066 -8.01613784669266e-14 0 0;-0.0006 -7.97097423623454e-14 0 0;-0.00054 -7.92173252807049e-14 0 0;-0.00048 -7.8684379151683e-14 0 0;-0.00042 -7.81111766403668e-14 0.00970851252903187 0.000859746923910395;-0.00036 -7.74980110077529e-14 0.00967004660196138 0.00105660952162374;-0.0003 -7.68451959607088e-14 0.00962663330036741 0.00125293153838193;-0.00024 -7.61530654914752e-14 0.00957829483529724 0.00144861253221356;-0.00018 -7.54219737067894e-14 0.00952505593760279 0.00164355238910644;-0.00012 -7.46522946467173e-14 0.00946694384528787 0.00183765137422769;-6e-05 -7.38444220932882e-14 0.00940398828957269 0.00203081018294999]  x5=0.000616440308025359  V1=[4.327e-18 2.694e-07 2.694e-07;377 377 377;-0.06841 1.312 -0.2585]  V2=[4.095e-15 0.006804 0.006804;377 377 377;-0.7508 1.28 -0.2912]  I1=[2.296e-17 0.0001774 0.0001774;377 377 377;-2.081 -0.2552 -1.826]  I2=[2.168e-17 0.0001764 0.0001764;377 377 377;0.8233 2.744 1.174]  nHarmo=1  Measurements=None  Decoupling=off  VsMag0=0  VrMag0=0  VsAngle0=0  VrAngle0=0  IsMag0=0  IrMag0=0  IsAngle0=0  IrAngle0=0
      settings: LibrarySourceBlock=sps_lib/Power Grid Elements/Distributed Parameters Line
  North Network : Subsystem
  ORE-NAN 117 km3 : spsDistributedParametersLineLib/Distributed Parameters Line  Phases=3  Length=117  Frequency=60  Resistance=[0.01273 0.3864]/6  Inductance="[0.9337e-3  4.1264e-3]/6"  Capacitance=[12.74e-9 7.751e-9]*6  x1=[-0.00072 1.25031115881766e-12 0 0;-0.00066 1.24217821786657e-12 0 0;-0.0006 1.23340975558641e-12 0 0;-0.00054 1.2240102580845e-12 0 0;-0.00048 1.21398453431744e-12 0 0;-0.00042 1.20333771363077e-12 0.0718847256273727 -0.331069943640762;-0.00036 1.19207524313468e-12 0.0801701064361215 -0.330062548180282;-0.0003 1.18020288491719e-12 0.0884144707370444 -0.328886286621298;-0.00024 1.16772671309613e-12 0.0966136005610266 -0.327541760760958;-0.00018 1.15465311071154e-12 0.104763301081748 -0.326029658483538;-0.00012 1.14098876645997e-12 0.112859402761832 -0.324350753408501;-6e-05 1.12674067127244e-12 0.120897763486062 -0.322505904494709]  x2=[-0.00072 -5.2979066475037e-13 0 0;-0.00066 -5.87075368339395e-13 0 0;-0.0006 -6.44059713322071e-13 0 0;-0.00054 -7.00714545454557e-13 0 0;-0.00048 -7.57010879077872e-13 0 0;-0.00042 -8.12919911947498e-13 0.0164675508368521 -0.0548306360800849;-0.00036 -8.68413039969138e-13 0.0178343300884094 -0.0545604446418457;-0.0003 -9.23461871833103e-13 0.019191984967153 -0.0542623390719667;-0.00024 -9.78038243539824e-13 0.0205398208717603 -0.0539364718867656;-0.00018 -1.03211423280908e-12 0.0218771482244773 -0.0535830098059159;-0.00012 -1.08566217336556e-12 0.0232032828239195 -0.0532021336671493;-6e-05 -1.13865466909341e-12 0.0245175461951216 -0.0527940383337362]  x3=[-0.00072 6.36492419409716e-14 0 0;-0.00066 6.2004212468118e-14 0 0;-0.0006 6.03274604944596e-14 0 0;-0.00054 5.86198438772889e-14 0 0;-0.00048 5.68822362648205e-14 0 0;-0.00042 5.5115526649216e-14 0.0453260916835141 -0.00163522208830896;-0.00036 5.332061891176e-14 0.0452815982279828 -0.000720475247532768;-0.0003 5.1498431360417e-14 0.0452139378700905 0.000194640201692917;-0.00024 4.96498962600084e-14 0.0451231452261262 0.00110965606939488;-0.00018 4.77759593552485e-14 0.0450092667472844 0.00202410421654765;-0.00012 4.58775793868843e-14 0.0448723606958991 0.00293751679458209;-6e-05 4.39557276011856e-14 0.0447124971156359 0.00384942648474536]  x4=[-0.00072 -5.51133194854429e-14 0 0;-0.00066 -5.39662006486721e-14 0 0;-0.0006 -5.27914717064687e-14 0 0;-0.00054 -5.15897336718661e-14 0 0;-0.00048 -5.03616013762483e-14 0 0;-0.00042 -4.9107703154791e-14 -0.0440965212761709 -0.0069700831639695;-0.00036 -4.78286805249936e-14 -0.0438354372199854 -0.00787131080385594;-0.0003 -4.65251878584673e-14 -0.0435519261441324 -0.00876851133569002;-0.00024 -4.5197892046146e-14 -0.043246133098117 -0.0096612257351013;-0.00018 -4.38474721570928e-14 -0.0429182145313119 -0.0105489972729076;-0.00012 -4.2474619091076e-14 -0.0425683382129152 -0.011431371748786;-6e-05 -4.10800352250914e-14 -0.0421966831461163 -0.0123078977236502]  x5=0.000661683633385019  V1=[2.771e-15 0.004375 0.004375;377 377 377;-0.7831 1.268 -0.3032]  V2=[4.095e-15 0.006804 0.006804;377 377 377;-0.7678 1.269 -0.3016]  I1=[9.029e-18 6.296e-05 6.296e-05;377 377 377;-1.689 -0.005215 -1.576]  I2=[6.955e-18 6.141e-05 6.141e-05;377 377 377;0.2743 2.461 0.89]  nHarmo=1  Measurements=None  Decoupling=off  VsMag0=0  VrMag0=0  VsAngle0=0  VrAngle0=0  IsMag0=0  IrMag0=0  IsAngle0=0  IrAngle0=0
      settings: LibrarySourceBlock=sps_lib/Power Grid Elements/Distributed Parameters Line
  OSI 1 : spsThreePhaseVIMeasurementLib/Three-Phase V-I Measurement  VoltageMeasurement=phase-to-ground  SetLabelV=on  LabelV=Vabc_OSI1  Vpu=off  VpuLL=off  CurrentMeasurement=no  SetLabelI=off  LabelI=Iabc  Ipu=off  Pbase=100e6  Vbase=500e3  OutputType=Complex  PhasorSimulation=off  PSBequivalent=0
  OSI-MPO 187 km : spsDistributedParametersLineLib/Distributed Parameters Line  Phases=3  Length=187  Frequency=60  Resistance=[0.01273 0.3864]/6  Inductance="[0.9337e-3  4.1264e-3]/6"  Capacitance=[12.74e-9 7.751e-9]*6  x1=[-0.00108 -6.54549696606161e-12 0 0;-0.00102 -6.41303632993048e-12 0 0;-0.00096 -6.27729466591367e-12 0 0;-0.0009 -6.13834142195471e-12 0 0;-0.00084 -5.99624768910077e-12 0 0;-0.00078 -5.85108616513116e-12 0 0;-0.00072 -5.70293111736384e-12 0 0;-0.00066 -5.55185834465882e-12 -10.2602241700737 7.15980830823418;-0.0006 -5.39794513863813e-12 -10.4449653142995 7.02257988847939;-0.00054 -5.24127024414194e-12 -10.6243626212696 6.8817585870913;-0.00048 -5.08191381894132e-12 -10.7983243080071 6.73741645084978;-0.00042 -4.91995739272796e-12 -10.9667613724985 6.58962732785885;-0.00036 -4.75548382540212e-12 -11.1295876392293 6.43846682976469;-0.0003 -4.58857726467996e-12 -11.2867198032727 6.28401229307122;-0.00024 -4.41932310304204e-12 -11.4380774729102 6.12634273957343;-0.00018 -4.2478079340449e-12 -11.5835832107612 5.96553883592827;-0.00012 -4.07411950801823e-12 -11.7231625734015 5.80168285238417;-6e-05 -3.89834668717019e-12 -11.8567441494501 5.63485862069001]  x2=[-0.00108 -7.84561445660388e-12 0 0;-0.00102 -7.67126701967385e-12 0 0;-0.00096 -7.49299482078784e-12 0 0;-0.0009 -7.31088906729689e-12 0 0;-0.00084 -7.12504292786941e-12 0 0;-0.00078 -6.93555148482438e-12 0 0;-0.00072 -6.74251168548546e-12 0 0;-0.00066 -6.54602229258095e-12 -15.1617352905941 10.4839839732469;-0.0006 -6.34618383371497e-12 -15.4315996223466 10.2807967237232;-0.00054 -6.14309854993566e-12 -15.6935688625891 10.0723496286284;-0.00048 -5.9368703434268e-12 -15.9475089830177 9.85874933334797;-0.00042 -5.7276047243495e-12 -16.1932900631746 9.64010511973986;-0.00036 -5.51540875686124e-12 -16.4307863569175 9.41652885022383;-0.0003 -5.30039100433995e-12 -16.6598763567542 9.18813491055058;-0.00024 -5.08266147384086e-12 -16.8804428560076 8.95504015127987;-0.00018 -4.86233155981498e-12 -17.0923730087812 8.71736382799765;-0.00012 -4.63951398711753e-12 -17.2955583876928 8.47522754030267;-6e-05 -4.41432275333592e-12 -17.4898950393481 8.22875516959387]  x3=[-0.00108 -9.98891454855098e-14 0 0;-0.00102 -9.94706186068957e-14 0 0;-0.00096 -9.90012007217966e-14 0 0;-0.0009 -9.84811319930764e-14 0 0;-0.00084 -9.79106784975064e-14 0 0;-0.00078 -9.72901320896357e-14 0 0;-0.00072 -9.66198102524731e-14 0 0;-0.00066 -9.59000559350565e-14 0.12998666699327 0.44814357245185;-0.0006 -9.51312373769942e-14 0.114772569365219 0.452153681044005;-0.00054 -9.43137479200667e-14 0.0994997519699273 0.455932459458097;-0.00048 -9.34480058069856e-14 0.084176028662984 0.459477974401268;-0.00042 -9.2534453967413e-14 0.0688092393443826 0.462788411922558;-0.00036 -9.15735597913506e-14 0.053407245947484 0.465862078340962;-0.0003 -9.05658148900141e-14 0.0379779284167062 0.468697401111945;-0.00024 -8.9511734844316e-14 0.022529180675999 0.471292929631988;-0.00018 -8.84118589410849e-14 0.0070689065901666 0.473647335980738;-0.00012 -8.72667498971562e-14 -0.00839498407889574 0.475759415600404;-6e-05 -8.60769935714759e-14 -0.0238545797189818 0.477628087912026]  x4=[-0.00108 -3.11023621438644e-14 0 0;-0.00102 -2.96925071924499e-14 0 0;-0.00096 -2.82674610057012e-14 0 0;-0.0009 -2.68279526635795e-14 0 0;-0.00084 -2.53747186451514e-14 0 0;-0.00078 -2.39085024517937e-14 0 0;-0.00072 -2.24300542268032e-14 0 0;-0.00066 -2.09401303716106e-14 -0.634736225685666 -0.0196454666466593;-0.0006 -1.94394931587907e-14 -0.631095245695991 -0.030084876481803;-0.00054 -1.79289103420703e-14 -0.627131385717318 -0.040508894338234;-0.00048 -1.64091547635307e-14 -0.622846673733657 -0.0509121870958033;-0.00042 -1.48810039582077e-14 -0.618243301882831 -0.0612894322377053;-0.00036 -1.33452397562904e-14 -0.613323625334938 -0.071635320573576;-0.0003 -1.18026478831221e-14 -0.608090161087407 -0.0819445589557727;-0.00024 -1.0254017557209e-14 -0.602545586677249 -0.0922118729874462;-0.00018 -8.70014108644106e-15 -0.596692738811184 -0.10243200972102;-0.00012 -7.14181346273322e-15 -0.59053461191433 -0.112599740345694;-6e-05 -5.5798319552923e-15 -0.584074356598195 -0.122709862862604]  x5=0.00105756273028204  V1=[3.05e-13 0.3186 0.3186;377 377 377;-0.6471 -1.909 2.804]  V2=[3.793e-13 0.4417 0.4417;377 377 377;-0.6023 -1.906 2.806]  I1=[5.824e-16 0.002377 0.002377;377 377 377;-1.191 -2.924 1.788]  I2=[4.03e-16 0.002279 0.002279;377 377 377;-0.283 -1.078 -2.649]  nHarmo=1  Measurements=None  Decoupling=off  VsMag0=0  VrMag0=0  VsAngle0=0  VrAngle0=0  IsMag0=0  IrMag0=0  IsAngle0=0  IrAngle0=0
      settings: LibrarySourceBlock=sps_lib/Power Grid Elements/Distributed Parameters Line
  PSS : Constant
  PSS_Equation : Subsystem
  Regulators 10 : Subsystem
  South Network : Subsystem
  Step : Step  Time=0.5  SampleTime=0.3
  Three-Phase Fault : spsThreePhaseFaultLib/Three-Phase Fault  InitialStates=0  FaultA=on  FaultB=on  FaultC=on  GroundFault=on  SwitchTimes="[1/60  5/60]"  External=on  SwitchStatus=NaN  FaultResistance=0.001  GroundResistance=0.01  SnubberResistance=1e6  SnubberCapacitance=inf  Measurements=None
  powergui : sps_lib/powergui  Priority=1  SimulationMode=Discrete  SampleTime=6e-5  frequency=60  Iterations=50  frequencyindice=60  Pbase=100e6  ErrMax=1e-4  UnitsV=kV  UnitsW=MW  buscounter=0  FunctionMessages=off  echomessages=off  EnableUseOfTLC=off  CurrentSourceSwitches=off  DisableSnubberDevices=off  DisableRonSwitches=off  DisableVfSwitches=off  DisplayEquations=off  AutomaticDiscreteSolvers=off  SolverType=Tustin/Backward Euler (TBE)  Interpol=off  ExternalGateDelay=off  methode=off  Ts=100  x0status=blocks  SPID=on  SwTol=0  HookPort=off  NonlinearTolerance=1e-4  nMaxIteration=100  ContinueOnMaxIteration=off  RestoreLinks=warning  ResistiveCurrentMeasurement=off  Frange=[0:2:500]  Ylog=off  Xlog=on  ShowGrid=off  save=off  variable=ZData  structure=0  ZoomFFT=off  StartTime=0.0  cycles=1  DisplayStyle=1  fundamental=60  FreqAxis=off  MaxFrequency=1000  frequencyindicesteady=1  RmsSteady=1  display=off
  wires:
  PSS/1 -> PSS_Equation/1(In1)
  Regulators 10/1(Pm) -> MPP10 3000 MVA 17KV/1
  MPP10 3000 MVA 17KV/1 -> Regulators 10/1(m)
  Regulators 10/2(Vf) -> MPP10 3000 MVA 17KV/2
  Step/1 -> Three-Phase Fault/1
  connections:
  South Network/LConn3 -- CON-OSI 144 km/RConn3
  South Network/LConn2 -- CON-OSI 144 km/RConn2
  South Network/LConn1 -- CON-OSI 144 km/RConn1
  OSI 1/LConn1 -- CON-OSI 144 km/LConn1
  CON-OSI 144 km/LConn2 -- OSI 1/LConn2
  CON-OSI 144 km/LConn3 -- OSI 1/LConn3
  Cs OSIS/LConn1 -- OSI 1/RConn1
  Cs OSIS/LConn2 -- OSI 1/RConn2
  Cs OSIS/LConn3 -- OSI 1/RConn3
  150 MW/LConn1 -- MPP10 3000 MVA 17KV/RConn1 -- "3000 MVA 17KV :650KV Transformer "/LConn1 -- Load Flow Bus1/LConn1
  150 MW/LConn2 -- "3000 MVA 17KV :650KV Transformer "/LConn2 -- MPP10 3000 MVA 17KV/RConn2
  "3000 MVA 17KV :650KV Transformer "/LConn3 -- MPP10 3000 MVA 17KV/RConn3 -- 150 MW/LConn3
  North Network/RConn1 -- ATL-MPO 350 km/RConn1
  Cs OSIS/RConn1 -- Load Flow Bus3/LConn1 -- OSI-MPO 187 km/LConn1
  Cs OSIS/RConn2 -- OSI-MPO 187 km/LConn2
  Cs OSIS/RConn3 -- OSI-MPO 187 km/LConn3
  MPP10-MPO 234 km/LConn1 -- 330 MVar/LConn1 -- "3000 MVA 17KV :650KV Transformer "/RConn1
  MPP10-MPO 234 km/LConn2 -- 330 MVar/LConn2 -- "3000 MVA 17KV :650KV Transformer "/RConn2
  MPP10-MPO 234 km/LConn3 -- "3000 MVA 17KV :650KV Transformer "/RConn3 -- 330 MVar/LConn3
  MPP10-MPO 234 km/RConn1 -- Cs MPOD/RConn1 -- Load Flow Bus2/LConn1 -- " Wind Generation + Load"/LConn1 -- OSI-MPO 187 km/RConn1
  MPP10-MPO 234 km/RConn2 -- " Wind Generation + Load"/LConn2 -- OSI-MPO 187 km/RConn2 -- Cs MPOD/RConn2
  MPP10-MPO 234 km/RConn3 -- " Wind Generation + Load"/LConn3 -- OSI-MPO 187 km/RConn3 -- Cs MPOD/RConn3
  MPO 3/RConn1 -- ATL-MPO 350 km/LConn1 -- Cs MPOD/LConn1
  MPO 3/RConn2 -- ATL-MPO 350 km/LConn2 -- Cs MPOD/LConn2
  MPO 3/RConn3 -- ATL-MPO 350 km/LConn3 -- Cs MPOD/LConn3
  NAN 1/LConn2 -- Three-Phase Fault/LConn2 -- MTL Load/LConn2 -- Home Network Load （with circuit breaker)/LConn2 -- NAN-SAT 109 km/RConn2 -- MPO-NAN 277 km/RConn2
  MTL Load/LConn1 -- Home Network Load （with circuit breaker)/LConn1 -- Load Flow Bus4/LConn1 -- NAN-SAT 109 km/RConn1 -- MPO-NAN 277 km/RConn1 -- NAN 1/LConn1 -- Three-Phase Fault/LConn1 -- Load Flow Bus5/LConn1
  ATL-MPO 350 km/RConn2 -- North Network/RConn2
  North Network/RConn3 -- ATL-MPO 350 km/RConn3
  North Network/LConn1 -- ORE-NAN 117 km3/LConn1
  North Network/LConn2 -- ORE-NAN 117 km3/LConn2
  North Network/LConn3 -- ORE-NAN 117 km3/LConn3
  NAN 1/RConn3 -- ORE-NAN 117 km3/RConn3
  ORE-NAN 117 km3/RConn2 -- NAN 1/RConn2
  ORE-NAN 117 km3/RConn1 -- NAN 1/RConn1
  South Network/LConn4 -- NAN-SAT 109 km/LConn1
  South Network/LConn5 -- NAN-SAT 109 km/LConn2
  South Network/LConn6 -- NAN-SAT 109 km/LConn3
  MPO-NAN 277 km/LConn3 -- 660 MVar/LConn3 -- MPO 3/LConn3
  MPO 3/LConn2 -- 660 MVar/LConn2 -- MPO-NAN 277 km/LConn2
  MPO-NAN 277 km/LConn1 -- 660 MVar/LConn1 -- MPO 3/LConn1
  MPO-NAN 277 km/RConn3 -- NAN-SAT 109 km/RConn3 -- Home Network Load （with circuit breaker)/LConn3 -- MTL Load/LConn3 -- Three-Phase Fault/LConn3 -- NAN 1/LConn3
